simulink model "generic_IVS"  (R2024a)
settings: Solver=FixedStepDiscrete  StartTime=0.0  StopTime=inf  FixedStep=0.001  RelTol=1e-3  EnableMultiTasking=on
undefined symbols (not defined in the file): filtered_route_waypoint_raw, route1_waypoint_x, route1_waypoint_y, route2_waypoint_raw, route2_waypoint_x, route2_waypoint_y, route3_waypoint_x, route3_waypoint_y, route4_waypoint_x, route4_waypoint_y, route5_waypoint_x, route5_waypoint_y
libraries: CarMaker4SL x125, slpidlib x7, simulink x1, robotalgslib x1
(part 4 of 5)

== system generic_IVS/CarMaker/Subsystem/Final Project/Scenario 1/Tollgate/Traffic_frenet1 ==
  Traffic info : Inport
  waypoint : Inport  Port=2
  MATLAB Function1 : MATLAB Function  TreatAsAtomicUnit=on
  MATLAB Function7 : MATLAB Function  TreatAsAtomicUnit=on
  MATLAB Function9 : MATLAB Function  TreatAsAtomicUnit=on
  Reshape : Reshape  OutputDimensionality=Customize  OutputDimensions=[8,8]
  Terminator1 : Terminator
  Terminator2 : Terminator
  Transpose : Math  Operator=transpose
  frenet_traffic_s : Outport
  frenet_traffic_d : Outport  Port=2
  wires:
  Reshape/1 -> Transpose/1
  MATLAB Function7/1(frenet_traffic) -> MATLAB Function1/1(frenet_traffics), MATLAB Function9/1(frenet_traffics)
  MATLAB Function7/3(num_vehicles) -> Terminator1/1
  MATLAB Function7/2(obs_sd) -> Terminator2/1
  Traffic info/1 -> Reshape/1
  Transpose/1 -> MATLAB Function7/1(traffic_data)
  MATLAB Function9/1(frenet_traffic_s) -> frenet_traffic_s/1
  waypoint/1 -> MATLAB Function7/2(waypoint)
  MATLAB Function1/1(frenet_traffic_s) -> frenet_traffic_d/1

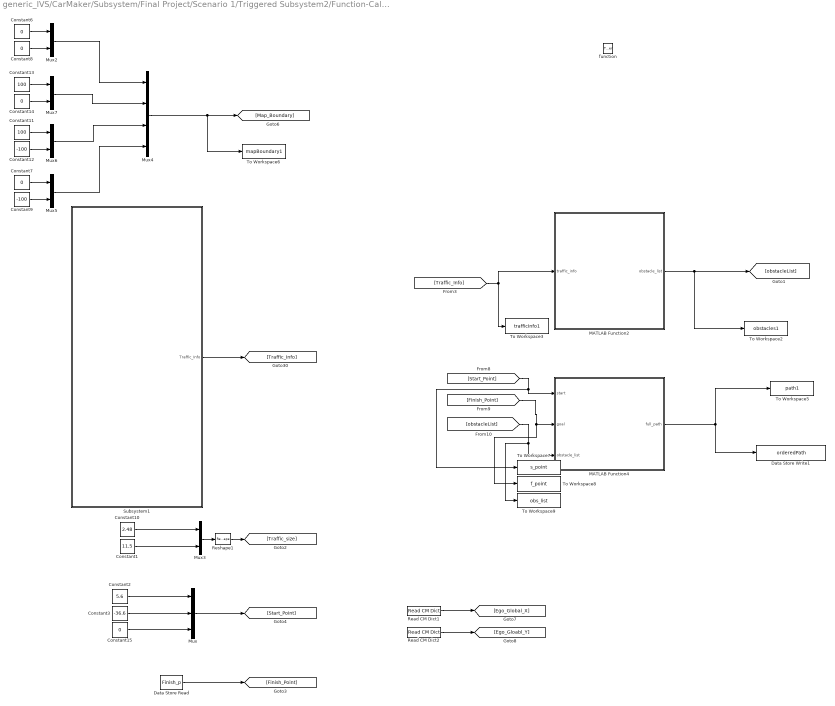
== system generic_IVS/CarMaker/Subsystem/Final Project/Scenario 1/Triggered Subsystem2/Function-Call Subsystem ==
  function : TriggerPort  TriggerType=function-call  VariantControl=(inherit)
  Constant1 : Constant  Value=11.5
  Constant10 : Constant  Value=2.48
  Constant11 : Constant  Value=100
  Constant12 : Constant  Value=-100
  Constant13 : Constant  Value=100
  Constant{6..8,14..15} (5 alike) : Constant  Value=0
  Constant2 : Constant  Value=5.6
  Constant3 : Constant  Value=-36.6
  Constant9 : Constant  Value=-100
  Data Store Read : DataStoreRead  DataStoreName=Finish_p  IndexOptions=Index vector (dialog)  Indices=1  OutputSizes=1
  Data Store Write1 : DataStoreWrite  DataStoreName=orderedPath  IndexOptions=Index vector (dialog)  Indices=1  OutputSizes=1
  MATLAB Function2 : MATLAB Function  TreatAsAtomicUnit=on
  MATLAB Function4 : MATLAB Function  TreatAsAtomicUnit=on
  Mux : Mux  Inputs=3
  Mux{2..3,5..7} (5 alike) : Mux  Inputs=2
  Mux4 : Mux
  Read CM Dict1 : CarMaker4SL/Read CM Dict  xname=Car.Fr1.tx  xsync=off  xstime=Inherited
  Read CM Dict2 : CarMaker4SL/Read CM Dict  xname=Car.Fr1.ty  xsync=off  xstime=Inherited
  Reshape1 : Reshape  OutputDimensionality=Row vector (2-D)  OutputDimensions=[2,2]
  Subsystem1 : Subsystem
  To Workspace2 : ToWorkspace  VariableName=obstacles1  SampleTime=-1
  To Workspace3 : ToWorkspace  VariableName=trafficInfo1  SampleTime=-1
      settings: Save2DSignal=2-D array (concatenate along first dimension)
  To Workspace5 : ToWorkspace  VariableName=path1  SampleTime=-1
      settings: Save2DSignal=2-D array (concatenate along first dimension)
  To Workspace6 : ToWorkspace  VariableName=mapBoundary1  SampleTime=-1
  To Workspace7 : ToWorkspace  VariableName=s_point  SampleTime=-1
      settings: Save2DSignal=2-D array (concatenate along first dimension)
  To Workspace8 : ToWorkspace  VariableName=f_point  SampleTime=-1
      settings: Save2DSignal=2-D array (concatenate along first dimension)
  To Workspace9 : ToWorkspace  VariableName=obs_list  SampleTime=-1
      settings: Save2DSignal=2-D array (concatenate along first dimension)
  wires:
  MATLAB Function4/1(full_path) -> To Workspace5/1, Data Store Write1/1
  [obstacleList] -> To Workspace9/1, MATLAB Function4/3(obstacle_list)
  [Finish_Point] -> MATLAB Function4/2(goal), To Workspace8/1
  [Start_Point] -> MATLAB Function4/1(start), To Workspace7/1
  Data Store Read/1 -> [Finish_Point]
  Constant3/1 -> Mux/2
  Mux/1 -> [Start_Point]
  Constant15/1 -> Mux/3
  Constant2/1 -> Mux/1
  Constant12/1 -> Mux6/2
  MATLAB Function2/1(obstacle_list) -> [obstacleList], To Workspace2/1
  Mux5/1 -> Mux4/4
  Mux4/1 -> [Map_Boundary], To Workspace6/1
  [Traffic_Info] -> MATLAB Function2/1(traffic_info), To Workspace3/1
  Constant13/1 -> Mux7/1
  Reshape1/1 -> [Traffic_size]
  Constant1/1 -> Mux3/2
  Constant6/1 -> Mux2/1
  Constant8/1 -> Mux2/2
  Constant10/1 -> Mux3/1
  Mux6/1 -> Mux4/3
  Mux3/1 -> Reshape1/1
  Constant7/1 -> Mux5/1
  Constant14/1 -> Mux7/2
  Constant11/1 -> Mux6/1
  Mux2/1 -> Mux4/1
  Mux7/1 -> Mux4/2
  Constant9/1 -> Mux5/2
  Subsystem1/1(Traffic_Info) -> [Traffic_Info]
  Read CM Dict1/1 -> [Ego_Global_X]
  Read CM Dict2/1 -> [Ego_Gloabl_Y]

== system generic_IVS/CarMaker/Subsystem/Final Project/Scenario 1/Triggered Subsystem2/Function-Call Subsystem1 ==
  function : TriggerPort  TriggerType=function-call  VariantControl=(inherit)
  Constant1 : Constant  Value=2
  Data Store Read2 : DataStoreRead  DataStoreName=orderedPath  IndexOptions=Index vector (dialog)  Indices=1  OutputSizes=1
  Data Store Read3 : DataStoreRead  DataStoreName=Finish_p  IndexOptions=Index vector (dialog)  Indices=1  OutputSizes=1
  MATLAB Function : MATLAB Function  TreatAsAtomicUnit=on
  MATLAB Function2 : MATLAB Function  TreatAsAtomicUnit=on
  Mux2 : Mux  Inputs=3
  Mux4 : Mux  Inputs=3
  Read CM Dict1 : CarMaker4SL/Read CM Dict  xname=Car.Fr1.tx  xsync=off  xstime=Inherited
  Read CM Dict2 : CarMaker4SL/Read CM Dict  xname=Car.Fr1.ty  xsync=off  xstime=Inherited
  Read CM Dict3 : CarMaker4SL/Read CM Dict  xname=Car.Fr1.rz  xsync=off  xstime=Inherited
  Read CM Dict4 : CarMaker4SL/Read CM Dict  xname=Car.v  xsync=off  xstime=Inherited
  Scope5 : Scope  NumInputPorts=2
  Scope6 : Scope
  Terminator2 : Terminator
  Write CM Dict3 : CarMaker4SL/Write CM Dict  xname=Car.CFL.rz_ext  xsync=off
  Write CM Dict4 : CarMaker4SL/Write CM Dict  xname=Car.CFR.rz_ext  xsync=off
  Write CM Dict6 : CarMaker4SL/Write CM Dict  xname=AccelCtrl.DesiredAx  xsync=off
  wires:
  Data Store Read3/1 -> [Finish_Point]
  [Ego_Vx] -> MATLAB Function/2(v), Scope5/1
  MATLAB Function2/3(target_velocity) -> [Target_Veolcity]  "targetV"
  [Ego_Yaw] -> Mux4/3
  [Ego_Global_X] -> Mux4/1
  [Ego_Gloabl_Y] -> Mux4/2
  Mux4/1 -> MATLAB Function2/1(currPoseRear)
  Constant1/1 -> [Target_Velocity]
  MATLAB Function2/1(DesiredAx) -> Write CM Dict6/1, Scope6/1  "acc"
  [Ego_Vx] -> MATLAB Function2/2(ego_v)  "egoV"
  [Target_Velocity] -> MATLAB Function2/3("target_velocity ")
  [Finish_Point] -> MATLAB Function2/4(goalPose)
  Data Store Read2/1 -> MATLAB Function/3(waypoints)
  [Ego_Global_X] -> Mux2/1
  Mux2/1 -> MATLAB Function/1(currPoseRear)
  [Ego_Yaw] -> Mux2/3
  [Ego_Gloabl_Y] -> Mux2/2
  MATLAB Function/1(delta) -> Write CM Dict4/1, Write CM Dict3/1
  Read CM Dict2/1 -> [Ego_Gloabl_Y]
  Read CM Dict1/1 -> [Ego_Global_X]
  Read CM Dict3/1 -> [Ego_Yaw]
  Read CM Dict4/1 -> [Ego_Vx]
  MATLAB Function2/2(stopFlag) -> Terminator2/1

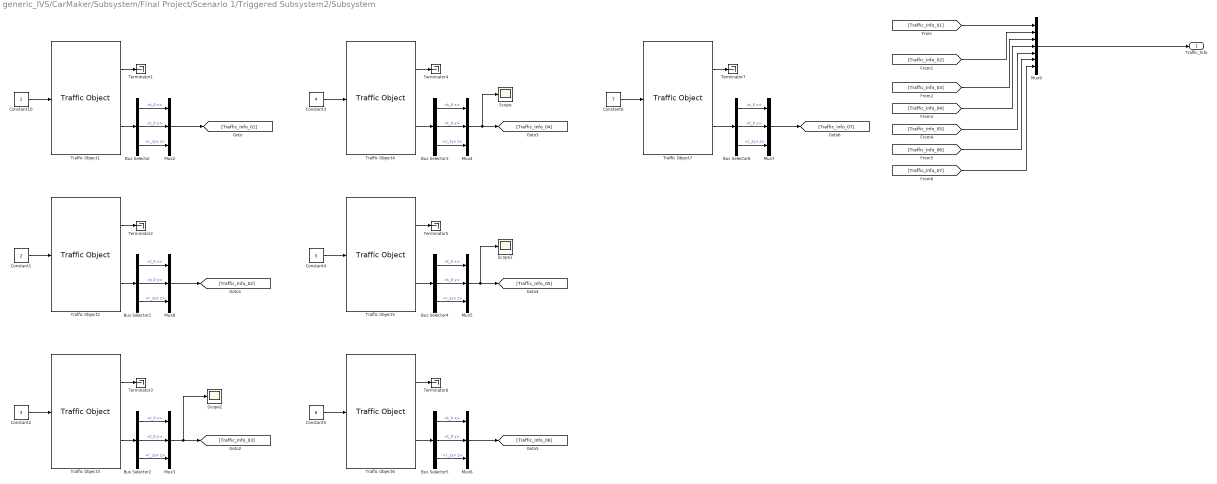
== system generic_IVS/CarMaker/Subsystem/Final Project/Scenario 1/Triggered Subsystem2/Subsystem ==
  Bus Selector{,1..6} (7 alike) : BusSelector  OutputSignals=t_0 x,t_0 y,r_zyx z
  Constant1 : Constant  Value=2
  Constant10 : Constant
  Constant2 : Constant  Value=3
  Constant3 : Constant  Value=4
  Constant4 : Constant  Value=5
  Constant5 : Constant  Value=6
  Constant6 : Constant  Value=7
  Mux{2..8} (7 alike) : Mux  Inputs=3
  Mux9 : Mux  Inputs=7
  Scope : Scope
  Scope1 : Scope
  Scope2 : Scope
  Terminator{1..7} (7 alike) : Terminator
  Traffic Object1 : CarMaker4SL/Traffic Object  xname=T01  ximode=Traffic Id  xstime=Inherited
      settings: SourceProductName=CarMaker4SL
  Traffic Object2 : CarMaker4SL/Traffic Object  xname=T02  ximode=Traffic Id  xstime=Inherited
      settings: SourceProductName=CarMaker4SL
  Traffic Object3 : CarMaker4SL/Traffic Object  xname=T03  ximode=Traffic Id  xstime=Inherited
      settings: SourceProductName=CarMaker4SL
  Traffic Object4 : CarMaker4SL/Traffic Object  xname=T04  ximode=Traffic Id  xstime=Inherited
      settings: SourceProductName=CarMaker4SL
  Traffic Object5 : CarMaker4SL/Traffic Object  xname=T05  ximode=Traffic Id  xstime=Inherited
      settings: SourceProductName=CarMaker4SL
  Traffic Object6 : CarMaker4SL/Traffic Object  xname=T06  ximode=Traffic Id  xstime=Inherited
      settings: SourceProductName=CarMaker4SL
  Traffic Object7 : CarMaker4SL/Traffic Object  xname=T07  ximode=Traffic Id  xstime=Inherited
      settings: SourceProductName=CarMaker4SL
  Traffic_Info : Outport
  wires:
  [Traffic_Info_07] -> Mux9/7
  [Traffic_Info_06] -> Mux9/6
  [Traffic_Info_05] -> Mux9/5
  [Traffic_Info_04] -> Mux9/4
  [Traffic_Info_03] -> Mux9/3
  Mux9/1 -> Traffic_Info/1
  [Traffic_Info_02] -> Mux9/2
  [Traffic_Info_01] -> Mux9/1
  Mux2/1 -> [Traffic_Info_01]
  Traffic Object7/2 -> Bus Selector6/1
  Bus Selector6/3 -> Mux7/3  "<r_zyx z>"
  Bus Selector6/1 -> Mux7/1  "<t_0 x>"
  Mux7/1 -> [Traffic_Info_07]
  Bus Selector6/2 -> Mux7/2  "<t_0 y>"
  Traffic Object6/2 -> Bus Selector5/1
  Bus Selector5/3 -> Mux6/3  "<r_zyx z>"
  Bus Selector5/1 -> Mux6/1  "<t_0 x>"
  Mux6/1 -> [Traffic_Info_06]
  Bus Selector5/2 -> Mux6/2  "<t_0 y>"
  Traffic Object5/2 -> Bus Selector4/1
  Bus Selector4/3 -> Mux5/3  "<r_zyx z>"
  Bus Selector4/1 -> Mux5/1  "<t_0 x>"
  Mux5/1 -> [Traffic_Info_05], Scope1/1
  Bus Selector4/2 -> Mux5/2  "<t_0 y>"
  Traffic Object4/2 -> Bus Selector3/1
  Bus Selector3/3 -> Mux4/3  "<r_zyx z>"
  Bus Selector3/1 -> Mux4/1  "<t_0 x>"
  Mux4/1 -> [Traffic_Info_04], Scope/1
  Bus Selector3/2 -> Mux4/2  "<t_0 y>"
  Traffic Object3/2 -> Bus Selector2/1
  Bus Selector2/3 -> Mux3/3  "<r_zyx z>"
  Bus Selector2/1 -> Mux3/1  "<t_0 x>"
  Mux3/1 -> [Traffic_Info_03], Scope2/1
  Bus Selector2/2 -> Mux3/2  "<t_0 y>"
  Traffic Object2/2 -> Bus Selector1/1
  Bus Selector1/3 -> Mux8/3  "<r_zyx z>"
  Bus Selector1/1 -> Mux8/1  "<t_0 x>"
  Mux8/1 -> [Traffic_Info_02]
  Bus Selector1/2 -> Mux8/2  "<t_0 y>"
  Bus Selector/3 -> Mux2/3  "<r_zyx z>"
  Bus Selector/2 -> Mux2/2  "<t_0 y>"
  Bus Selector/1 -> Mux2/1  "<t_0 x>"
  Traffic Object1/2 -> Bus Selector/1
  Traffic Object7/1 -> Terminator7/1
  Constant6/1 -> Traffic Object7/1
  Constant5/1 -> Traffic Object6/1
  Traffic Object6/1 -> Terminator6/1
  Traffic Object5/1 -> Terminator5/1
  Constant4/1 -> Traffic Object5/1
  Constant3/1 -> Traffic Object4/1
  Traffic Object4/1 -> Terminator4/1
  Traffic Object3/1 -> Terminator3/1
  Constant2/1 -> Traffic Object3/1
  Constant1/1 -> Traffic Object2/1
  Traffic Object2/1 -> Terminator2/1
  Traffic Object1/1 -> Terminator1/1
  Constant10/1 -> Traffic Object1/1

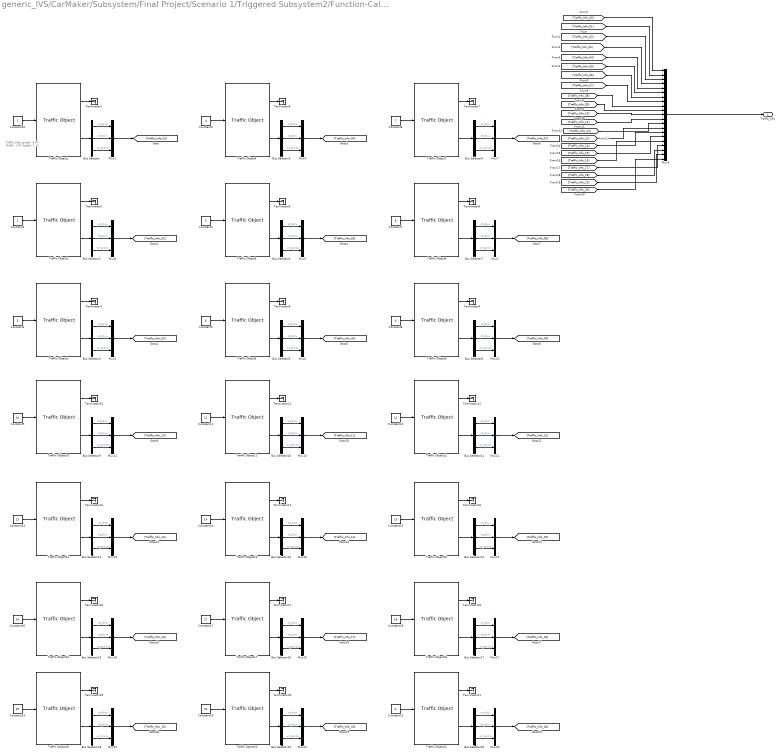
== system generic_IVS/CarMaker/Subsystem/Final Project/Scenario 1/Triggered Subsystem2/Function-Call Subsystem/Subsystem1 ==
  note: Traffic Size
      | Length: 4.47
      | Width: 1.97
      | Height: 1.12
  Bus Selector{,1..20} (21 alike) : BusSelector  OutputSignals=t_0 x,t_0 y,r_zyx z
  Constant1 : Constant  Value=2
  Constant10 : Constant
  Constant11 : Constant  Value=11
  Constant12 : Constant  Value=12
  Constant13 : Constant  Value=13
  Constant14 : Constant  Value=14
  Constant15 : Constant  Value=15
  Constant16 : Constant  Value=16
  Constant17 : Constant  Value=17
  Constant18 : Constant  Value=18
  Constant19 : Constant  Value=19
  Constant2 : Constant  Value=3
  Constant20 : Constant  Value=20
  Constant21 : Constant  Value=0
  Constant3 : Constant  Value=4
  Constant4 : Constant  Value=5
  Constant5 : Constant  Value=6
  Constant6 : Constant  Value=7
  Constant7 : Constant  Value=8
  Constant8 : Constant  Value=9
  Constant9 : Constant  Value=10
  Mux{1..8,10..22} (21 alike) : Mux  Inputs=3
  Mux9 : Mux  Inputs=21
  Terminator{1..21} (21 alike) : Terminator
  Traffic Object1 : CarMaker4SL/Traffic Object  xname=T01  ximode=Traffic Id  xstime=Inherited
      settings: SourceProductName=CarMaker4SL
  Traffic Object10 : CarMaker4SL/Traffic Object  xname=T10  ximode=Traffic Id  xstime=Inherited
      settings: SourceProductName=CarMaker4SL
  Traffic Object11 : CarMaker4SL/Traffic Object  xname=T11  ximode=Traffic Id  xstime=Inherited
      settings: SourceProductName=CarMaker4SL
  Traffic Object12 : CarMaker4SL/Traffic Object  xname=T12  ximode=Traffic Id  xstime=Inherited
      settings: SourceProductName=CarMaker4SL
  Traffic Object13 : CarMaker4SL/Traffic Object  xname=T13  ximode=Traffic Id  xstime=Inherited
      settings: SourceProductName=CarMaker4SL
  Traffic Object14 : CarMaker4SL/Traffic Object  xname=T14  ximode=Traffic Id  xstime=Inherited
      settings: SourceProductName=CarMaker4SL
  Traffic Object15 : CarMaker4SL/Traffic Object  xname=T15  ximode=Traffic Id  xstime=Inherited
      settings: SourceProductName=CarMaker4SL
  Traffic Object16 : CarMaker4SL/Traffic Object  xname=T16  ximode=Traffic Id  xstime=Inherited
      settings: SourceProductName=CarMaker4SL
  Traffic Object17 : CarMaker4SL/Traffic Object  xname=T17  ximode=Traffic Id  xstime=Inherited
      settings: SourceProductName=CarMaker4SL
  Traffic Object18 : CarMaker4SL/Traffic Object  xname=T18  ximode=Traffic Id  xstime=Inherited
      settings: SourceProductName=CarMaker4SL
  Traffic Object19 : CarMaker4SL/Traffic Object  xname=T19  ximode=Traffic Id  xstime=Inherited
      settings: SourceProductName=CarMaker4SL
  Traffic Object2 : CarMaker4SL/Traffic Object  xname=T02  ximode=Traffic Id  xstime=Inherited
      settings: SourceProductName=CarMaker4SL
  Traffic Object20 : CarMaker4SL/Traffic Object  xname=T20  ximode=Traffic Id  xstime=Inherited
      settings: SourceProductName=CarMaker4SL
  Traffic Object21 : CarMaker4SL/Traffic Object  xname=T00  ximode=Traffic Id  xstime=Inherited
      settings: SourceProductName=CarMaker4SL
  Traffic Object3 : CarMaker4SL/Traffic Object  xname=T03  ximode=Traffic Id  xstime=Inherited
      settings: SourceProductName=CarMaker4SL
  Traffic Object4 : CarMaker4SL/Traffic Object  xname=T04  ximode=Traffic Id  xstime=Inherited
      settings: SourceProductName=CarMaker4SL
  Traffic Object5 : CarMaker4SL/Traffic Object  xname=T05  ximode=Traffic Id  xstime=Inherited
      settings: SourceProductName=CarMaker4SL
  Traffic Object6 : CarMaker4SL/Traffic Object  xname=T06  ximode=Traffic Id  xstime=Inherited
      settings: SourceProductName=CarMaker4SL
  Traffic Object7 : CarMaker4SL/Traffic Object  xname=T07  ximode=Traffic Id  xstime=Inherited
      settings: SourceProductName=CarMaker4SL
  Traffic Object8 : CarMaker4SL/Traffic Object  xname=T08  ximode=Traffic Id  xstime=Inherited
      settings: SourceProductName=CarMaker4SL
  Traffic Object9 : CarMaker4SL/Traffic Object  xname=T09  ximode=Traffic Id  xstime=Inherited
      settings: SourceProductName=CarMaker4SL
  Traffic_Info : Outport
  wires:
  Constant10/1 -> Traffic Object1/1
  Traffic Object1/1 -> Terminator1/1
  Traffic Object2/1 -> Terminator2/1
  Constant1/1 -> Traffic Object2/1
  Constant2/1 -> Traffic Object3/1
  Traffic Object3/1 -> Terminator3/1
  Traffic Object4/1 -> Terminator4/1
  Constant3/1 -> Traffic Object4/1
  Constant4/1 -> Traffic Object5/1
  Traffic Object5/1 -> Terminator5/1
  Traffic Object6/1 -> Terminator6/1
  Constant5/1 -> Traffic Object6/1
  Constant6/1 -> Traffic Object7/1
  Traffic Object7/1 -> Terminator7/1
  [Traffic_Info_04] -> Mux9/5
  [Traffic_Info_05] -> Mux9/6
  [Traffic_Info_06] -> Mux9/7
  [Traffic_Info_07] -> Mux9/8
  Traffic Object1/2 -> Bus Selector/1
  Bus Selector/1 -> Mux2/1  "<t_0 x>"
  Bus Selector/2 -> Mux2/2  "<t_0 y>"
  Bus Selector/3 -> Mux2/3  "<r_zyx z>"
  Bus Selector1/2 -> Mux8/2  "<t_0 y>"
  Mux8/1 -> [Traffic_Info_02]
  Bus Selector1/1 -> Mux8/1  "<t_0 x>"
  Bus Selector1/3 -> Mux8/3  "<r_zyx z>"
  Traffic Object2/2 -> Bus Selector1/1
  Bus Selector2/2 -> Mux3/2  "<t_0 y>"
  Mux3/1 -> [Traffic_Info_03]
  Bus Selector2/1 -> Mux3/1  "<t_0 x>"
  Bus Selector2/3 -> Mux3/3  "<r_zyx z>"
  Traffic Object3/2 -> Bus Selector2/1
  Bus Selector3/2 -> Mux4/2  "<t_0 y>"
  Mux4/1 -> [Traffic_Info_04]
  Bus Selector3/1 -> Mux4/1  "<t_0 x>"
  Bus Selector3/3 -> Mux4/3  "<r_zyx z>"
  Traffic Object4/2 -> Bus Selector3/1
  Bus Selector4/2 -> Mux5/2  "<t_0 y>"
  Mux5/1 -> [Traffic_Info_05]
  Bus Selector4/1 -> Mux5/1  "<t_0 x>"
  Bus Selector4/3 -> Mux5/3  "<r_zyx z>"
  Traffic Object5/2 -> Bus Selector4/1
  Bus Selector5/2 -> Mux6/2  "<t_0 y>"
  Mux6/1 -> [Traffic_Info_06]
  Bus Selector5/1 -> Mux6/1  "<t_0 x>"
  Bus Selector5/3 -> Mux6/3  "<r_zyx z>"
  Traffic Object6/2 -> Bus Selector5/1
  Bus Selector6/2 -> Mux7/2  "<t_0 y>"
  Mux7/1 -> [Traffic_Info_07]
  Bus Selector6/1 -> Mux7/1  "<t_0 x>"
  Bus Selector6/3 -> Mux7/3  "<r_zyx z>"
  Traffic Object7/2 -> Bus Selector6/1
  Mux2/1 -> [Traffic_Info_01]
  [Traffic_Info_01] -> Mux9/2
  [Traffic_Info_02] -> Mux9/3
  Mux9/1 -> Traffic_Info/1
  [Traffic_Info_03] -> Mux9/4
  Traffic Object8/1 -> Terminator8/1
  Bus Selector7/2 -> Mux1/2  "<t_0 y>"
  Mux1/1 -> [Traffic_Info_08]
  Bus Selector7/3 -> Mux1/3  "<r_zyx z>"
  Traffic Object8/2 -> Bus Selector7/1
  Constant7/1 -> Traffic Object8/1
  Bus Selector7/1 -> Mux1/1  "<t_0 x>"
  Traffic Object9/1 -> Terminator9/1
  Bus Selector8/2 -> Mux10/2  "<t_0 y>"
  Mux10/1 -> [Traffic_Info_09]
  Bus Selector8/3 -> Mux10/3  "<r_zyx z>"
  Traffic Object9/2 -> Bus Selector8/1
  Constant8/1 -> Traffic Object9/1
  Bus Selector8/1 -> Mux10/1  "<t_0 x>"
  Bus Selector10/1 -> Mux13/1  "<t_0 x>"
  Traffic Object12/1 -> Terminator12/1
  Bus Selector11/2 -> Mux11/2  "<t_0 y>"
  Bus Selector11/3 -> Mux11/3  "<r_zyx z>"
  Mux11/1 -> [Traffic_Info_12]
  Bus Selector11/1 -> Mux11/1  "<t_0 x>"
  Bus Selector9/3 -> Mux12/3  "<r_zyx z>"
  Mux12/1 -> [Traffic_Info_10]
  Traffic Object10/2 -> Bus Selector9/1
  Constant9/1 -> Traffic Object10/1
  Traffic Object11/1 -> Terminator11/1
  Bus Selector9/1 -> Mux12/1  "<t_0 x>"
  Mux13/1 -> [Traffic_Info_11]
  Bus Selector10/3 -> Mux13/3  "<r_zyx z>"
  Constant11/1 -> Traffic Object11/1
  Traffic Object11/2 -> Bus Selector10/1
  Traffic Object12/2 -> Bus Selector11/1
  Traffic Object10/1 -> Terminator10/1
  Constant12/1 -> Traffic Object12/1
  Bus Selector9/2 -> Mux12/2  "<t_0 y>"
  Bus Selector10/2 -> Mux13/2  "<t_0 y>"
  Bus Selector13/1 -> Mux16/1  "<t_0 x>"
  Traffic Object15/1 -> Terminator15/1
  Bus Selector14/2 -> Mux14/2  "<t_0 y>"
  Bus Selector14/3 -> Mux14/3  "<r_zyx z>"
  Mux14/1 -> [Traffic_Info_15]
  Bus Selector14/1 -> Mux14/1  "<t_0 x>"
  Bus Selector12/3 -> Mux15/3  "<r_zyx z>"
  Mux15/1 -> [Traffic_Info_13]
  Traffic Object13/2 -> Bus Selector12/1
  Constant13/1 -> Traffic Object13/1
  Traffic Object14/1 -> Terminator14/1
  Bus Selector12/1 -> Mux15/1  "<t_0 x>"
  Mux16/1 -> [Traffic_Info_14]
  Bus Selector13/3 -> Mux16/3  "<r_zyx z>"
  Constant14/1 -> Traffic Object14/1
  Traffic Object14/2 -> Bus Selector13/1
  Traffic Object15/2 -> Bus Selector14/1
  Traffic Object13/1 -> Terminator13/1
  Constant15/1 -> Traffic Object15/1
  Bus Selector12/2 -> Mux15/2  "<t_0 y>"
  Bus Selector13/2 -> Mux16/2  "<t_0 y>"
  Bus Selector16/1 -> Mux19/1  "<t_0 x>"
  Traffic Object18/1 -> Terminator18/1
  Bus Selector17/2 -> Mux17/2  "<t_0 y>"
  Bus Selector17/3 -> Mux17/3  "<r_zyx z>"
  Mux17/1 -> [Traffic_Info_18]
  Bus Selector17/1 -> Mux17/1  "<t_0 x>"
  Bus Selector15/3 -> Mux18/3  "<r_zyx z>"
  Mux18/1 -> [Traffic_Info_16]
  Traffic Object16/2 -> Bus Selector15/1
  Constant16/1 -> Traffic Object16/1
  Traffic Object17/1 -> Terminator17/1
  Bus Selector15/1 -> Mux18/1  "<t_0 x>"
  Mux19/1 -> [Traffic_Info_17]
  Bus Selector16/3 -> Mux19/3  "<r_zyx z>"
  Constant17/1 -> Traffic Object17/1
  Traffic Object17/2 -> Bus Selector16/1
  Traffic Object18/2 -> Bus Selector17/1
  Traffic Object16/1 -> Terminator16/1
  Constant18/1 -> Traffic Object18/1
  Bus Selector15/2 -> Mux18/2  "<t_0 y>"
  Bus Selector16/2 -> Mux19/2  "<t_0 y>"
  Bus Selector19/2 -> Mux22/2  "<t_0 y>"
  Bus Selector18/2 -> Mux21/2  "<t_0 y>"
  Traffic Object20/1 -> Terminator20/1
  Traffic Object19/1 -> Terminator19/1
  Traffic Object21/2 -> Bus Selector20/1
  Bus Selector19/3 -> Mux22/3  "<r_zyx z>"
  Constant21/1 -> Traffic Object21/1
  Traffic Object20/2 -> Bus Selector19/1
  Mux22/1 -> [Traffic_Info_20]
  Traffic Object19/2 -> Bus Selector18/1
  Bus Selector18/3 -> Mux21/3  "<r_zyx z>"
  Bus Selector20/2 -> Mux20/2  "<t_0 y>"
  Bus Selector18/1 -> Mux21/1  "<t_0 x>"
  Mux20/1 -> [Traffic_Info_00]
  Constant19/1 -> Traffic Object19/1
  Constant20/1 -> Traffic Object20/1
  Bus Selector20/3 -> Mux20/3  "<r_zyx z>"
  Mux21/1 -> [Traffic_Info_19]
  Bus Selector19/1 -> Mux22/1  "<t_0 x>"
  Bus Selector20/1 -> Mux20/1  "<t_0 x>"
  Traffic Object21/1 -> Terminator21/1
  [Traffic_Info_00] -> Mux9/1
  [Traffic_Info_08] -> Mux9/9
  [Traffic_Info_09] -> Mux9/10
  [Traffic_Info_10] -> Mux9/11
  [Traffic_Info_11] -> Mux9/12
  [Traffic_Info_12] -> Mux9/13
  [Traffic_Info_13] -> Mux9/14
  [Traffic_Info_14] -> Mux9/15
  [Traffic_Info_15] -> Mux9/16
  [Traffic_Info_16] -> Mux9/17
  [Traffic_Info_17] -> Mux9/18
  [Traffic_Info_18] -> Mux9/19
  [Traffic_Info_19] -> Mux9/20
  [Traffic_Info_20] -> Mux9/21

== matlab function generic_IVS/CarMaker/Subsystem/Final Project/Scenario 1/Drive/MATLAB Function7 ==
  settings: updateMethod=DISCRETE
  data: poly_coeff input; lateral_error output; velocity input; lookahead_time input; x_lookahead output
function [lateral_error, x_lookahead] = compute_lateral_error(poly_coeff, velocity, lookahead_time)
    % === 이전 에러 저장용 ===
    persistent prev_error
    if isempty(prev_error)
        prev_error = 0;
    end

    % Lookahead 지점 계산
    x_lookahead = velocity * lookahead_time + 2.9;

    % 경로 상의 lookahead 지점에서의 y값 계산
    y_desired = polyval(poly_coeff, x_lookahead);

    % 초기 계산된 lateral error
    raw_error = y_desired;

    % === 급격한 튐 보정 ===
    MAX_DELTA = 0.5;  % 프레임 간 최대 허용 변화량 (단위: m)
    delta = raw_error - prev_error;
    if abs(delta) > MAX_DELTA
        % 제한된 변화량만 반영
        lateral_error = prev_error + sign(delta) * MAX_DELTA;
    else
        lateral_error = raw_error;
    end

    % 상태 갱신
    prev_error = lateral_error;
end

== matlab function generic_IVS/CarMaker/Subsystem/Final Project/Scenario 1/Triggered Subsystem2/Function-Call Subsystem1/MATLAB Function ==
  data: currPoseRear input; v input; waypoints input; delta output
function delta = lateral_spp_controller(currPoseRear, v, waypoints)
%▴ Hybrid Stanley & Pure Pursuit + Monotonic Index Enforcement
% Inputs:
%   currPoseRear : [x_rear; y_rear; psi] (후륜축 기준 위치 및 자세)
%   v            : 현재 속도 (m/s)
%   waypoints    : N×3 [x_i, y_i, psi_i] (경로 웨이포인트)
% Output:
%   delta        : 전륜 조향각 (rad)

    %#codegen
    %% persistent 변수 초기화
    persistent idx_last delta_prev
    if isempty(idx_last)
        idx_last   = 1;    % 마지막 타겟 인덱스 (초기값)
    end
    if isempty(delta_prev)
        delta_prev = 0;    % 이전 조향각 (로우패스 필터용)
    end

    %% 파라미터
    L        = 2.9;                             % 휠베이스 [m]
    k_st     = 1.4;                             % Stanley 이득
    eps_v    = 0.1;                             % 속도 안정화 상수
    deltaMax = deg2rad(37);                     % 최대 조향각 제한 ±40°
    e_thresh = 0.2;                             % SPP 전환 임계값 [m]
    k_pp     = 0.3;                             % 룩어헤드 속도 이득
    Ld_min   = 2.0;                             % 룩어헤드 최솟값 [m]
    Ld_max   = 5.0;                             % 룩어헤드 최댓값 [m]
    alpha_f  = 0.3;                            % 로우패스 필터 상수

    %% 전륜축 위치 계산 (후륜축 기준 → 전륜축 좌표 변환)
    x_f = currPoseRear(1) + L*cos(currPoseRear(3));
    y_f = currPoseRear(2) + L*sin(currPoseRear(3));

    %% 전방 웨이포인트만 선별 (로컬 좌표계)
    psi_wrapped = wrapToPi(currPoseRear(3));    % yaw를 –π~π로 유지
    heading_vec = [cos(psi_wrapped), sin(psi_wrapped)];
    diffs       = waypoints(:,1:2) - currPoseRear(1:2)';
    forward_idx = find(diffs * heading_vec' > 0);  % 전방 idx
    if isempty(forward_idx)
        forward_idx = (1:size(waypoints,1))';       % 전방이 없으면 전체 사용
    end

    %% 룩어헤드 거리 계산
    Ld_raw = k_pp * v + eps_v;
    Ld     = min(max(Ld_raw, Ld_min), Ld_max);

    %% 후보 인덱스 범위 설정 (룩어헤드 윈도우)
    N = size(waypoints,1);
    extra     = round(0.2 * Ld);                  % 윈도우 여분
    start_idx = max(idx_last - extra, 1);
    end_idx   = min(idx_last + round(Ld) + extra, N);
    cand_idx  = intersect(forward_idx, (start_idx:end_idx)');

    if isempty(cand_idx)
        cand_idx = forward_idx;  % 후보 없으면 전방 전체 사용
    end

    %% 최단거리 웨이포인트 선택
    dists = hypot(waypoints(cand_idx,1)-x_f, waypoints(cand_idx,2)-y_f);
    [~, rel] = min(dists);
    idx_new  = cand_idx(rel);  % 새로 계산된 인덱스

    %% 1) Monotonic Index Enforcement 적용
    % 새 인덱스(idx_new)가 이전 idx_last보다 작으면 무시
    if idx_new < idx_last
        idx_last = idx_last;    % 변경 없이 유지
    else
        idx_last = idx_new;     % 증가 시에만 갱신
    end

    %% 참조점 정보 추출
    x_ref   = waypoints(idx_last,1);
    y_ref   = waypoints(idx_last,2);
    psi_ref = waypoints(idx_last,3);

    %% Heading error 및 Cross-Track error 계산
    theta_e = wrapToPi(psi_ref - currPoseRear(3));  
    e_cte   = -(x_f - x_ref)*sin(psi_ref) + (y_f - y_ref)*cos(psi_ref);

    %% 제어 분기: Pure Pursuit vs Stanley
    if abs(e_cte) > e_thresh
        % Pure Pursuit
        alpha     = wrapToPi(atan2(y_ref-currPoseRear(2), x_ref-currPoseRear(1)) ...
                     - currPoseRear(3));
        delta_cmd = atan2(2 * L * sin(alpha), Ld);
    else
        % Stanley
        delta_cmd = theta_e + atan((k_st * e_cte) / (v + eps_v));
    end

    %% 로우패스 필터 적용 및 조향각 포화
    delta       = alpha_f * delta_cmd + (1 - alpha_f) * delta_prev;
    delta_prev  = delta;  
    delta       = max(min(delta, deltaMax), -deltaMax);

end

== matlab function generic_IVS/CarMaker/Subsystem/Final Project/Scenario 1/PreParking/MATLAB Function4  ==
  settings: sampleTime=0.05
  data: waypoints input; local_waypoints_ output; vehicle_position input; head input
function local_waypoints_ = global_to_local_waypoints(waypoints, vehicle_position, head)
    % 글로벌 좌표를 로컬 좌표로 변환해주는 함수
    % waypoints : Global_Waypoints [id, X, Y]
    % vehicle_position : [Ego_Global_X, Ego_Global_Y]
    % head : Ego_Yaw (rad)
    % 출력: Local Waypoints

    % 초기화
    num_points = size(waypoints, 1);
    local_waypoints_ = NaN(num_points, 2);  % [x_local, y_local]

    % 차량 위치 추출
    ego_x = vehicle_position(1);
    ego_y = vehicle_position(2);
    ego_yaw = head;

    % 회전 행렬 생성 (글로벌→로컬 변환)
    R = [cos(-ego_yaw) -sin(-ego_yaw); 
         sin(-ego_yaw)  cos(-ego_yaw)];

    count = 0;
    % 각 웨이포인트에 대해 변환 수행
    for i = 1:num_points
        % 글로벌 좌표에서 차량까지의 상대 위치
        dx = waypoints(i, 1) - ego_x;  % X 좌표 차이
        dy = waypoints(i, 2) - ego_y;  % Y 좌표 차이

        % 회전 변환 적용
        local_pos = R * [dx; dy];
        distance = sqrt(dx.^2 + dy.^2); % 차량으로부터 waypoint까지의 길이 계산

        % 시작 좌표 저장
        if count == 0 && local_pos(1) > 0 && distance < 15
            count = count + 1;
            local_waypoints_(count, :) = [local_pos(1) local_pos(2)];     % 로컬 x 좌표 
        end

        % 아래의 조건을 모두 만족하는 경우에만 좌표 저장
        % 1. x 좌표가 0보다 큰 경우
        % 2. x의 현재 좌표가 이전 x의 좌표보다 큰 경우
        % 3. 차량으로부터 waypoint까지의 길이가 30m 이내인 경우 (길이는 임의로 테스트 한 후 설정 가능할 듯)
        if count  ~= 0 && local_pos(1) > 0 && local_pos(1) > local_waypoints_(count, 1)  && distance < 15
            count = count + 1;
            local_waypoints_(count, :) = [local_pos(1) local_pos(2)];
        end
    end
end

== matlab function generic_IVS/CarMaker/Subsystem/Final Project/Scenario 1/PreParking/MATLAB Function7 ==
  settings: sampleTime=0.05
  data: local_waypoints input; poly_coeff output
function poly_coeff = fit_polynomial_to_waypoints(local_waypoints)
    % waypoint를 curve fitting 한 다항식 계수 반환
    % input: 로컬 좌표 웨이포인트
    % output: 다항식 계수 (3차)

    % 웨이포인트 추출
    x_points = local_waypoints(:, 1);  % 로컬 x 좌표
    y_points = local_waypoints(:, 2);  % 로컬 y 좌표

    % 유효한 웨이포인트만 사용 (x 좌표가 양수인 것만)
    valid_indices = x_points > 0;
    x_valid = x_points(valid_indices);
    y_valid = y_points(valid_indices);
    poly_coeff = polyfit(x_valid, y_valid, 3);
end

== matlab function generic_IVS/CarMaker/Subsystem/Final Project/Scenario 1/Triggered Subsystem2/Function-Call Subsystem1/MATLAB Function2 ==
  settings: sampleTime=0.05
  data: currPoseRear input; DesiredAx output; ego_v input; target_velocity input; goalPose input; stopFlag output; target_velocity output
function [DesiredAx,stopFlag,target_velocity] = longitudinal_goal_controller(currPoseRear, ego_v,target_velocity,goalPose)
%▴ 종방향 속도 제어 및 목표 도달 확인
% Inputs:
%   currPoseRear: [x_rear; y_rear; psi] (후륜축 기준)
%   v           : 속도 (m/s)
%   goalPose    : [x_goal; y_goal; psi_goal]
% Outputs:
%   DesiredAx   : 원하는 가속도 (m/s^2)
%   stopFlag    : 목표 도달 시 true

    persistent Kp Kd dt prev_error
  if isempty(Kp)
    % — PD 게인 설정 (필요에 따라 조정하세요) —
    Kp = 1.8;    % 비례 이득
    Kd = 0.1;    % 미분 이득
    % — 제어 업데이트 주기 (Simulink 샘플타임과 동일하게) —
    dt = 0.05;    % [s]
    % — previous error 초기화 —
    prev_error = target_velocity - ego_v;
  end

  % 1) 속도 오차
  error = target_velocity - ego_v;
  % 2) 오차 변화율 (미분항)
  derivative = (error - prev_error) / dt;
  % 3) PD 제어 법칙
  DesiredAx = Kp * error + Kd * derivative;
  % 4) 이전 오차 갱신
  prev_error = error;


    %#codegen
    % 1) 위치·헤딩 오차 계산
    dx     = currPoseRear(1) - goalPose(1);
    dy     = currPoseRear(2) - goalPose(2);
    dist   = hypot(dx, dy);                                           % 거리 계산 :contentReference[oaicite:3]{index=3}
    yawErr = wrapToPi(goalPose(3) - currPoseRear(3));                 % –π~π 범위 :contentReference[oaicite:4]{index=4}

    % 2) 목표 도달 여부 판단 (Goal Checking in Parking Valet) :contentReference[oaicite:5]{index=5}
    posTol = 4.5;             % 위치 허용 오차 [m]
    yawTol = deg2rad(40);     % 헤딩 허용 오차 [rad]
    almostFlag = dist<9;
    distFlag = dist <= posTol;
    yawFlag = abs(yawErr) <= yawTol;
    stopFlag = distFlag && yawFlag;

    % 3) DesiredAx 계산
    if stopFlag
        DesiredAx = -1000;
        disp("stopFlag")% 도착 시 완전 정지
    elseif almostFlag
        target_velocity = 1.5;
        disp("almost goal")% 근접 시 제동 가속도
        error      = target_velocity - ego_v;
        derivative = (error - prev_error)/dt;
        DesiredAx  = Kp*error + Kd*derivative;
        prev_error = error;
    end
end

== matlab function generic_IVS/CarMaker/Subsystem/Final Project/Scenario 1/Drive/MATLAB Function2 ==
  settings: updateMethod=DISCRETE
  data: local_waypoints input; poly_coeff output
function poly_coeff = fit_polynomial_to_waypoints(local_waypoints)
    % waypoint를 curve fitting 한 다항식 계수 반환
    % input: 로컬 좌표 웨이포인트
    % output: 다항식 계수 (3차)

    % 웨이포인트 추출
    x_points = local_waypoints(:, 1);  % 로컬 x 좌표
    y_points = local_waypoints(:, 2);  % 로컬 y 좌표

    % 유효한 웨이포인트만 사용 (x 좌표가 양수인 것만)
    valid_indices = x_points > 0;
    x_valid = x_points(valid_indices);
    y_valid = y_points(valid_indices);
    poly_coeff = polyfit(x_valid, y_valid, 3);
end

== matlab function generic_IVS/CarMaker/Subsystem/Final Project/Scenario 1/Tollgate/MATLAB Function1 ==
  data: poly_coeff input; lateral_error output; velocity input; lookahead_time input; x_lookahead output
function [lateral_error, x_lookahead] = compute_lateral_error(poly_coeff, velocity, lookahead_time)
    % Lookahead 지점 계산
    x_lookahead = velocity * lookahead_time + 2.9;

    % 경로 상의 lookahead 지점에서의 y값 계산
    y_desired = polyval(poly_coeff, x_lookahead);

    % subplot(122);
    % x_fit = linspace(0, length(x_lookahead));
    % y_fit = polyval(poly_coeff, x_fit);
    % plot(x_fit, y_fit);

    % lateral error : 차량 y=0 위치와 경로 y_desired의 차이
    lateral_error = y_desired;
end

== matlab function generic_IVS/CarMaker/Subsystem/Final Project/Scenario 1/Tollgate/MATLAB Function3 ==
  data: local_waypoints input; poly_coeff output
function poly_coeff = fit_polynomial_to_waypoints(local_waypoints)
    % waypoint를 curve fitting 한 다항식 계수 반환
    % input: 로컬 좌표 웨이포인트
    % output: 다항식 계수 (3차)

    % 웨이포인트 추출
    x_points = local_waypoints(:, 1);  % 로컬 x 좌표
    y_points = local_waypoints(:, 2);  % 로컬 y 좌표

    % 유효한 웨이포인트만 사용 (x 좌표가 양수인 것만)
    valid_indices = x_points > 0;
    x_valid = x_points(valid_indices);
    y_valid = y_points(valid_indices);
    poly_coeff = polyfit(x_valid, y_valid, 3);
    
    % subplot(121);
    % scatter(local_waypoints(:, 1), local_waypoints(:, 2));
end

== matlab function generic_IVS/CarMaker/Subsystem/Final Project/Scenario 1/Tollgate/MATLAB Function4  ==
  settings: sampleTime=0.05
  data: waypoints input; local_waypoints_ output; vehicle_position input; head input; toll_num input
function local_waypoints_ = global_to_local_waypoints(waypoints, vehicle_position, head, toll_num)
    % 글로벌 좌표를 로컬 좌표로 변환해주는 함수
    % waypoints : Global_Waypoints [id, X, Y]
    % vehicle_position : [Ego_Global_X, Ego_Global_Y]
    % head : Ego_Yaw (rad)
    % 출력: Local Waypoints

    % 초기화
    num_points = size(waypoints, 1);
    local_waypoints_ = NaN(num_points, 2);  % [x_local, y_local]
    
    offset = 0;
    switch toll_num
        case 1
            offset = 3.5;
        case 2
            offset = 0;
        case 3
            offset = -3.5;
    end

    % 차량 위치 추출
    ego_x = vehicle_position(1);
    ego_y = vehicle_position(2);
    ego_yaw = head;

    % 회전 행렬 생성 (글로벌→로컬 변환)
    R = [cos(-ego_yaw) -sin(-ego_yaw); 
         sin(-ego_yaw)  cos(-ego_yaw)];

    count = 0;
    % 각 웨이포인트에 대해 변환 수행
    for i = 1:num_points
        % 글로벌 좌표에서 차량까지의 상대 위치
        dx = waypoints(i, 1) - ego_x;  % X 좌표 차이
        dy = waypoints(i, 2) - ego_y;  % Y 좌표 차이

        % 회전 변환 적용
        local_pos = R * [dx; dy];
        distance = sqrt(dx.^2 + dy.^2); % 차량으로부터 waypoint까지의 길이 계산
        
        if vehicle_position(2) < -80
            % 시작 좌표 저장
            if count == 0 && local_pos(1) > 0 && distance < 15
                count = count + 1;
                local_waypoints_(count, :) = [local_pos(1), local_pos(2) + offset];     % 로컬 x 좌표 
            end
    
            % 아래의 조건을 모두 만족하는 경우에만 좌표 저장
            % 1. x 좌표가 0보다 큰 경우
            % 2. x의 현재 좌표가 이전 x의 좌표보다 큰 경우
            % 3. 차량으로부터 waypoint까지의 길이가 30m 이내인 경우 (길이는 임의로 테스트 한 후 설정 가능할 듯)
            if count  ~= 0 && local_pos(1) > 0 && local_pos(1) > local_waypoints_(count, 1)  && distance < 15
                count = count + 1;
                local_waypoints_(count, :) = [local_pos(1) , local_pos(2) + offset];
            end
        else
            % 시작 좌표 저장
            if count == 0 && local_pos(1) > 0 && distance < 15
                count = count + 1;
                local_waypoints_(count, :) = [local_pos(1), local_pos(2) - 3.5];     % 로컬 x 좌표 
            end
    
            % 아래의 조건을 모두 만족하는 경우에만 좌표 저장
            % 1. x 좌표가 0보다 큰 경우
            % 2. x의 현재 좌표가 이전 x의 좌표보다 큰 경우
            % 3. 차량으로부터 waypoint까지의 길이가 30m 이내인 경우 (길이는 임의로 테스트 한 후 설정 가능할 듯)
            if count  ~= 0 && local_pos(1) > 0 && local_pos(1) > local_waypoints_(count, 1)  && distance < 15
                count = count + 1;
                local_waypoints_(count, :) = [local_pos(1) , local_pos(2) - 3.5];
            end
        end
    end

end

== stateflow chart generic_IVS/CarMaker/Subsystem/Final Project/Scenario 1/Main_chart ==
  settings: updateMethod=DISCRETE  sampleTime=0.05
  state Driving
    en:
    send(driving);
    du:
    send(driving);
  state PassTollgate
    du:
    send(tollgate);
  state Parking
    du:
    send(parking);
  note: ##5.4  -> 30
      | ##4.4 - > 35
  state Ready2Parking
    du:
    send(ready2parking);
  state AngleConrol
    du:
    send(angleCon);
  (default) -> Driving
  Driving -> PassTollgate : [(global_X <= -105  &&  global_X >= -200) && (global_Y >= -170 && global_Y <= 30)]
  PassTollgate -> Ready2Parking : [(global_X<-79 && global_X >-95) && (global_Y>10)]
  AngleConrol -> Parking : [ (global_X >= 4.4) && (global_Y >= -40)]
  Ready2Parking -> AngleConrol : [(global_Y <= -28&& global_Y>= -40.0) && (global_X > -3)]
  data: global_X input; global_Y input
  events: ready2parking output FUNCTION_CALL_EVENT; driving output FUNCTION_CALL_EVENT; tollgate output FUNCTION_CALL_EVENT; parking output FUNCTION_CALL_EVENT; angleCon output FUNCTION_CALL_EVENT

== matlab function generic_IVS/CarMaker/Subsystem/Final Project/Scenario 1/Tollgate/Traffic_frenet1/MATLAB Function1 ==
  data: frenet_traffics input; frenet_traffic_s output
function frenet_traffic_s = fcn(frenet_traffics)

frenet_traffic_s = frenet_traffics(:,4);

== matlab function generic_IVS/CarMaker/Subsystem/Final Project/Scenario 1/Tollgate/Traffic_frenet1/MATLAB Function7 ==
  data: traffic_data input; frenet_traffic output; waypoint input; obs_sd output; num_vehicles output
function [frenet_traffic,obs_sd,num_vehicles]  = global2frenet_traffic(traffic_data, waypoint)
    % traffic_data : 8x7 행렬 (각 차량의 global X, Y, Yaw, Vx, Vy, Ax, Ay)
    % waypoint : 차선의 waypoint 정보 (nx2 행렬)
    % 반환 : 각 차량의 Frenet 좌표 [s, s_dot, s_dd, d, d_dot, d_dd]

    % 차량의 개수 (8대의 차량)
    num_vehicles = size(traffic_data, 1);
    
    % 결과 저장을 위한 행렬 초기화
    frenet_traffic = zeros(num_vehicles, 6);  % [s, s_dot, s_dd, d, d_dot, d_dd]
    
    % 각 차량에 대해 Frenet 좌표 계산
    for i = 1:num_vehicles
        % 각 차량의 global 좌표 정보
        x = traffic_data(i, 1);   % 차량의 global X
        y = traffic_data(i, 2);   % 차량의 global Y 
        Vx = traffic_data(i, 4);  % 차량의 longitudinal 속도
        Vy = traffic_data(i, 5);  % 차량의 lateral 속도
        Ax = traffic_data(i, 6);  % 차량의 longitudinal 가속도
        Ay = traffic_data(i, 7);  % 차량의 lateral 가속도
        yaw = traffic_data(i, 3); % 차량의 yaw (heading)

        % 1) 가장 가까운 waypoint를 찾기 위한 거리 계산
        dists = hypot(waypoint(:, 1) - x, waypoint(:, 2) - y);  % 차량과 waypoint 간의 거리
        [~, idx] = min(dists);  % 가장 가까운 waypoint 인덱스
        
        % 2) 이전, 다음 waypoint 인덱스 계산
        next_wp = idx;
        prev_wp = idx - 1;
        if prev_wp < 1
            prev_wp = length(waypoint);
        end
        
        % 3) 기준선 tangent, normal 벡터 계산
        dx = waypoint(next_wp, 1) - waypoint(prev_wp, 1);
        dy = waypoint(next_wp, 2) - waypoint(prev_wp, 2);
        seg_len = hypot(dx, dy);  % 세그먼트의 길이
        t = [dx; dy] / seg_len;   % tangent unit vector (차선 방향 벡터)
        n = [-t(2); t(1)];        % normal unit vector (법선 벡터)

        % 4) Frenet 위치 (s, d) 계산
        % 4-1) 기준선 시작점부터 prev_wp까지 누적 거리 계산
        s = 0;
        for j = 1:prev_wp-1
            s = s + hypot(waypoint(j+1, 1) - waypoint(j, 1), waypoint(j+1, 2) - waypoint(j, 2));
        end
        
        % 4-2) 차량-이전 waypoint 벡터 계산
        delta = [x - waypoint(prev_wp, 1); y - waypoint(prev_wp, 2)];
        
        % 4-3) 차량-이전 waypoint의 projection length (종방향 거리 s)
        proj = dot(delta, t);
        s = s + proj;  % 누적 거리 계산
        
        % 4-4) 차량-이전 waypoint의 lateral offset (횡방향 거리 d)
        d = dot(delta, n);

        % 5) 차량의 속도 및 가속도를 기준으로 Frenet 속도 및 가속도 계산
        % 5-1) 전역 속도 -> 차량 축 기준 속도 변환
        R = [cos(yaw), -sin(yaw); sin(yaw), cos(yaw)];  % 회전 행렬
        v_global = R * [Vx; Vy];  % 차량의 global 속도
        a_global = R * [Ax; Ay];  % 차량의 global 가속도

        % 5-2) Frenet 속도
        s_dot = dot(v_global, t);  % 종방향 속도
        d_dot = dot(v_global, n);  % 횡방향 속도

        % 5-3) Frenet 가속도
        s_dd = dot(a_global, t);  % 종방향 가속도
        d_dd = dot(a_global, n);  % 횡방향 가속도

        % 6) 결과 저장
        frenet_traffic(i, :) = [s, s_dot, s_dd, d, d_dot, d_dd];

        obs_sd = frenet_traffic(:, [1, 4]);
    end
end

== matlab function generic_IVS/CarMaker/Subsystem/Final Project/Scenario 1/Tollgate/Traffic_frenet1/MATLAB Function9 ==
  data: frenet_traffics input; frenet_traffic_s output
function frenet_traffic_s = fcn(frenet_traffics)

frenet_traffic_s = frenet_traffics(:,1);

== matlab function generic_IVS/CarMaker/Subsystem/Final Project/Scenario 1/Tollgate/Get frenet1/MATLAB Function ==
  settings: sampleTime=0.05
  data: x input; close_wp output; y input; mapx input; mapy input; min_len output
function [close_wp,min_len] = get_closest_waypoints(x, y, mapx, mapy)
% 입력:
%   x, y     : 현재 위치
%   mapx     : 지도 상의 x 좌표 배열
%   mapy     : 지도 상의 y 좌표 배열
% 출력:
%   close_wp : 가장 가까운 waypoint 인덱스

min_len = 1e10;
close_wp = 1; % MATLAB은 1-indexing

for i = 1:length(mapx)%200
    mx = mapx(i);
    my = mapy(i);
    dist = sqrt((x - mx)^2 + (y - my)^2);

    if dist < min_len
        min_len = dist;
        close_wp = i;
    end
end

% function [close_wp, min_len] = get_closest_waypoints(x, y, mapx, mapy)
% 
%     초기 탐색 범위 제한 (초반 튐 방지)
%     search_range = 1:min(300, length(mapx));
% 
%     min_len = Inf;
%     close_wp = 1;
% 
%     for i = search_range
%         mx = mapx(i);
%         my = mapy(i);
% 
%         dx = x - mx;
%         dy = y - my;
%         dist = hypot(dx, dy);
% 
%         진행 방향 고려 (다음 wp가 존재할 때만)
%         if i < length(mapx)
%             dx_map = mapx(i+1) - mx;
%             dy_map = mapy(i+1) - my;
%             dot_p = dx * dx_map + dy * dy_map;
% 
%             if dist < min_len && dot_p > 0
%                 min_len = dist;
%                 close_wp = i;
%             end
%         end
%     end
% 
%     최악의 경우 dot 조건 못 만족 → 그냥 최소 거리 반환
%     if isinf(min_len)
%         min_len = 1e10;
%         for i = search_range
%             mx = mapx(i);
%             my = mapy(i);
%             dist = hypot(x - mx, y - my);
%             if dist < min_len
%                 min_len = dist;
%                 close_wp = i;
%             end
%         end
%     end
% end

== matlab function generic_IVS/CarMaker/Subsystem/Final Project/Scenario 1/Tollgate/Get frenet1/MATLAB Function1 ==
  settings: sampleTime=0.05
  data: closest_wp input; x input; next_wp output; y input; mapx input; mapy input
function next_wp = next_waypoint(closest_wp, x, y, mapx, mapy)
% 현재 위치(x, y) 기준 가장 가까운 웨이포인트(closest_wp) 기준
% 다음 웨이포인트 index를 반환하는 함수

    % 예외 방지: map index 제한
    N = length(mapx);
    if closest_wp >= N
        next_wp = N;  % 맵 경계 조건 처리
        return;
    end

    % 맵 방향 벡터 (다음 웨이포인트 방향)
    dx_map = mapx(closest_wp + 1) - mapx(closest_wp);
    dy_map = mapy(closest_wp + 1) - mapy(closest_wp);
    map_vec = [dx_map, dy_map];

    % 차량 벡터
    dx_ego = x - mapx(closest_wp);
    dy_ego = y - mapy(closest_wp);
    ego_vec = [dx_ego, dy_ego];

    % 내적 → 진행 방향 판단
    dot_product = dx_map * dx_ego + dy_map * dy_ego;
    direction = sign(dot_product);

    % 다음 웨이포인트 결정
    if direction >= 0
        next_wp = min(closest_wp + 1, N);  % 경계 조건 보정
    else
        next_wp = closest_wp;
    end
end

== stateflow chart generic_IVS/CarMaker/Subsystem/Final Project/Scenario 1/Triggered Subsystem2/Chart1 ==
  settings: sampleTime=0.05
  state drawMap
    entry:
    draw_Map();
  state goParking
    during:
    go_Parking();
  (default) -> drawMap
  drawMap -> goParking : after(10,tick)
  events: go_Parking output FUNCTION_CALL_EVENT; draw_Map output FUNCTION_CALL_EVENT

== matlab function generic_IVS/CarMaker/Subsystem/Final Project/Scenario 1/Triggered Subsystem2/Function-Call Subsystem/MATLAB Function2 ==
  settings: sampleTime=0.1
  data: traffic_info input; obstacle_list output
function obstacle_list = add_obstacle_(traffic_info)
    % 차량 사이즈
    disp("Start adding obstacles")
    car_w = 1.97;            % 전폭
    car_l = 4.47;            % 전장

    % 장애물 파라미터
    r = car_w / 2 + 0.6;       % 각 원의 반지름 (1.24 + 2)
    n_circles = 5;          % 각 차량당 원 개수
    interval = car_l / n_circles;  % 원 간격

    % 최대 장애물 개수
    max_obs = 150;
    obstacle_list = zeros(max_obs, 3);  % [x, y, r]

    % === 데이터 복원 ===
    % 데이터가 직렬화된 벡터 형태로 들어오는 경우 처리
    if size(traffic_info, 2) == 1
        % 데이터를 3열 형태로 변환
        n = length(traffic_info) / 3;
        if mod(length(traffic_info), 3) == 0
            % 직렬 데이터를 [N x 3] 행렬로 변환
            latest_data = reshape(traffic_info, 3, n)';  % [N x 3]
            %disp('Reconstructed Data:');
            %disp(latest_data);  % 디버그 출력
        else
            warning('Invalid data length for traffic_info');
            return;
        end
    else
        latest_data = traffic_info;
    end

    % === 데이터 유효성 검사 ===
    if isempty(latest_data) || size(latest_data, 2) < 3
        warning('Latest data is empty or has incorrect dimensions');
        return;
    end

    % 중복 제거: unique 함수 사용 가능 여부 확인
    if size(latest_data, 1) > 1
        % unique 함수로 중복 좌표 제거
        [~, unique_indices] = unique(latest_data(:, 1:2), 'rows', 'stable');
        unique_data = latest_data(unique_indices, :);
    else
        % 데이터가 하나만 있는 경우 그대로 사용
        unique_data = latest_data;
    end

    % 입력 데이터 유효성 검사 및 reshape 처리
    unique_data = reshape(unique_data, [], 3);  % [N x 3]
    [n_rows, ~] = size(unique_data);

    % 장애물 좌표 생성
    count = 0;
    for i = 1:n_rows
        x_head = unique_data(i, 1);
        y_head = unique_data(i, 2);
        yaw = unique_data(i, 3);  % 각도(rad)

        % Yaw 값 검증
        if isnan(yaw) || ~isfinite(yaw)
            yaw = 0;
        end

        % 장애물 생성 (차량의 길이 방향으로)
        for j = 0:n_circles-1
            dx = cos(yaw) * (j * interval);
            dy = sin(yaw) * (j * interval);
            xc = x_head + dx;
            yc = y_head + dy;

            count = count + 1;
            if count <= max_obs
                obstacle_list(count, :) = [xc, yc, r];
            else
                break;
            end
        end
    end

    % 디버그: 결과 확인
    %disp('Generated Obstacle List:');
    %disp(obstacle_list);
end
